simulink model "angelbot_monitor"  (R2015b)
settings: Solver=ode5  StartTime=0.0  StopTime=inf  FixedStep=0.001  RelTol=1e-3
undefined symbols (not defined in the file or in its folder): Angular, Linear
libraries: robotlib x6, simulink x1
settings Model: Creator=weberhsu  LastModifiedBy=root

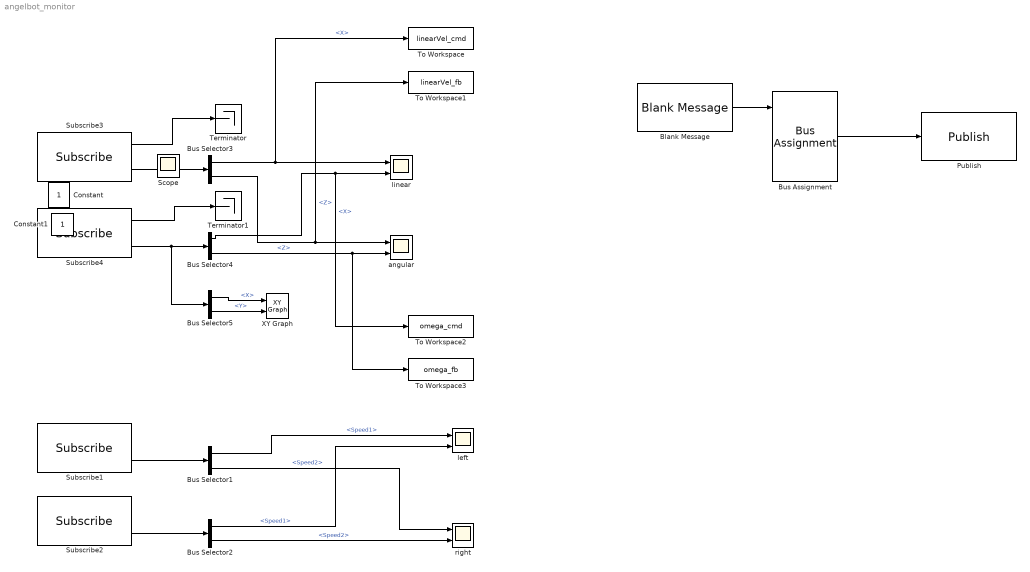
== system angelbot_monitor ==
  Blank Message : robotlib/Blank Message  SourceLibraryInfo=This block requires Robotics System Toolbox  messageType=geometry_msgs/Twist  SampleTime=inf
  Bus Assignment : BusAssignment  AssignedSignals=Linear.X,Angular.Z
  Bus Selector1 : BusSelector  OutputSignals=Speed1,Speed2
  Bus Selector2 : BusSelector  OutputSignals=Speed1,Speed2
  Bus Selector3 : BusSelector  OutputSignals=Linear.X,Angular.Z
  Bus Selector4 : BusSelector  OutputSignals=Twist.Twist.Linear.X,Twist.Twist.Angular.Z
  Bus Selector5 : BusSelector  OutputSignals=Pose.Pose.Position.X,Pose.Pose.Position.Y
  Publish : robotlib/Publish  SourceLibraryInfo=This block requires Robotics System Toolbox  topicSource=Select from ROS network  topic=/angelbot/cmd_vel  messageType=geometry_msgs/Twist  messageQueueLength=1
  Subscribe1 : robotlib/Subscribe  SourceLibraryInfo=This block requires Robotics System Toolbox  topicSource=Select from ROS network  topic=/cmd_wheel_angularVel  messageType=angelbot/WheelCmd  sampleTime=-1  messageQueueLength=1
  Subscribe2 : robotlib/Subscribe  SourceLibraryInfo=This block requires Robotics System Toolbox  topicSource=Select from ROS network  topic=/feedback_wheel_angularVel  messageType=angelbot/WheelFb  sampleTime=-1  messageQueueLength=1
  Subscribe3 : robotlib/Subscribe  SourceLibraryInfo=This block requires Robotics System Toolbox  topicSource=Select from ROS network  topic=/angelbot/cmd_vel  messageType=geometry_msgs/Twist  sampleTime=-1  messageQueueLength=1
  Subscribe4 : robotlib/Subscribe  SourceLibraryInfo=This block requires Robotics System Toolbox  topicSource=Select from ROS network  topic=/angelbot/odom  messageType=nav_msgs/Odometry  sampleTime=-1  messageQueueLength=1
  Terminator : Terminator
  Terminator1 : Terminator
  To Workspace : ToWorkspace  VariableName=linearVel_cmd  SaveFormat=Timeseries  SampleTime=-1
  To Workspace1 : ToWorkspace  VariableName=linearVel_fb  SaveFormat=Timeseries  SampleTime=-1
  To Workspace2 : ToWorkspace  VariableName=omega_cmd  SaveFormat=Timeseries  SampleTime=-1
  To Workspace3 : ToWorkspace  VariableName=omega_fb  SaveFormat=Timeseries  SampleTime=-1
  XY Graph : simulink/Sinks/XY Graph  xmin=-10  xmax=20  ymin=-10  ymax=20  st=-1
  angular : Scope  NumInputPorts=2
  left : Scope  NumInputPorts=2
  linear : Scope  NumInputPorts=2
  right : Scope  NumInputPorts=2
  Constant : Constant  IOType=siggen  VectorParams1D=off  SampleTime=1
  Constant1 : Constant  IOType=siggen
  Scope : Scope
  wires:
  Bus Selector1/2 -> right/1  "<Speed2>"
  Subscribe1/2 -> Bus Selector1/1
  Subscribe2/2 -> Bus Selector2/1
  Bus Selector1/1 -> left/1  "<Speed1>"
  Bus Selector2/1 -> left/2  "<Speed1>"
  Bus Selector2/2 -> right/2  "<Speed2>"
  Subscribe3/2 -> Bus Selector3/1
  Subscribe4/2 -> Bus Selector5/1, Bus Selector4/1
  Bus Selector3/1 -> To Workspace/1, linear/1  "<X>"
  Bus Selector4/1 -> To Workspace2/1, linear/2  "<X>"
  Bus Selector3/2 -> To Workspace1/1, angular/1  "<Z>"
  Bus Selector4/2 -> To Workspace3/1, angular/2  "<Z>"
  Blank Message/1 -> Bus Assignment/1
  Bus Assignment/1 -> Publish/1
  Subscribe3/1 -> Terminator/1
  Subscribe4/1 -> Terminator1/1
  Bus Selector5/1 -> XY Graph/1  "<X>"
  Bus Selector5/2 -> XY Graph/2  "<Y>"
